simulink library "avlAero2DCoeffs_ul"  (R2018b)
settings: Solver=VariableStepAuto  StartTime=0.0  StopTime=10.0  RelTol=1e-3
values from neighbouring files (symbols this model uses):
  k_CS_gain = calculate_2D_gains(dsgnTest_1,nom_a,nom_b,df,da,de,dr)    [avlAero2DCoeffs_ts.m]
undefined symbols (not defined in the file or in its folder): CDtot_2D_Tbl, CLtot_2D_Tbl, Cltot_2D_Tbl, Cmtot_2D_Tbl, Cntot_2D_Tbl
settings Model: Creator=mcobb  LastModifiedBy=asiddiq2

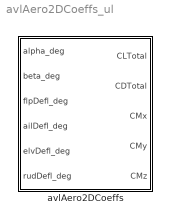
== system avlAero2DCoeffs_ul ==
  avlAero2DCoeffs : Subsystem  mask{CLTable=CLtot_2D_Tbl, CDTable=CDtot_2D_Tbl, CMxTable=Cltot_2D_Tbl, CMyTable=Cmtot_2D_Tbl, CMzTable=Cntot_2D_Tbl, CsGainMatrix=k_CS_gain}
      mask prompts: CLTable "CL lookup table object"; CDTable "CD lookup table object"; CMxTable "CMx lookup table object"; CMyTable "CMy lookup table object"; CMzTable "CMz lookup table object"; CsGainMatrix "Control surface gain matrix"

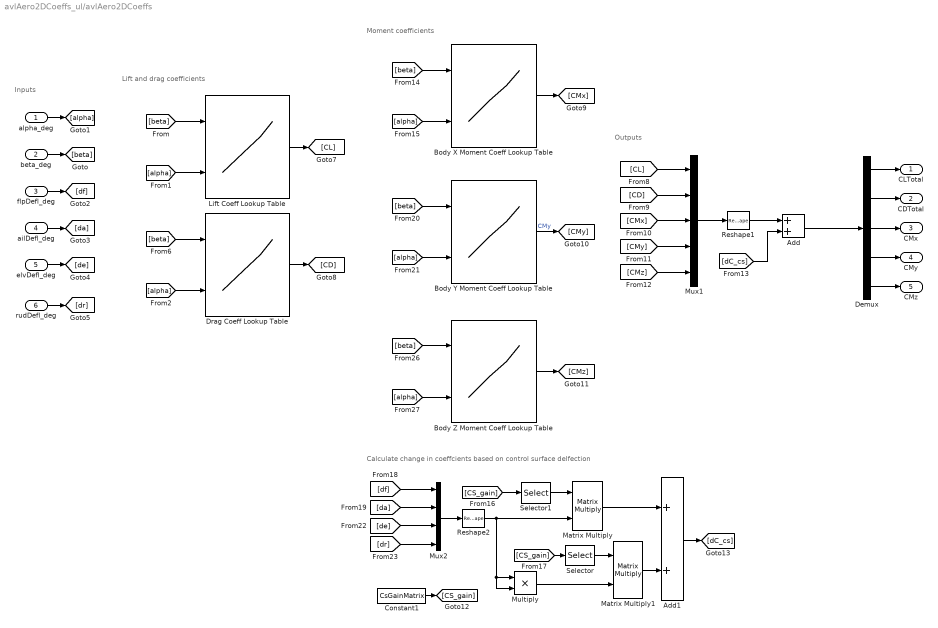
== system avlAero2DCoeffs_ul/avlAero2DCoeffs ==
  note: Outputs
  note: Inputs
  note: Lift and drag coefficients
  note: Moment coefficients
  note: Calculate change in coeffcients based on control surface
      | delfection
  alpha_deg : Inport
  beta_deg : Inport  Port=2
  flpDefl_deg : Inport  Port=3
  ailDefl_deg : Inport  Port=4
  elvDefl_deg : Inport  Port=5
  rudDefl_deg : Inport  Port=6
  Add : Sum
  Add1 : Sum
  Body X Moment Coeff Lookup Table : Lookup_n-D  DataSpecification=Lookup table object  LookupTableObject=CMxTable  BreakpointsForDimension3=[5, 7]  Table=reshape(repmat([4 5 6;16 19 20;10 18 23],1,2),[3,3,2])  InternalRulePriority=Speed  RndMeth=Simplest  InputSameDT=on
  Body Y Moment Coeff Lookup Table : Lookup_n-D  DataSpecification=Lookup table object  LookupTableObject=CMyTable  BreakpointsForDimension3=[5, 7]  Table=reshape(repmat([4 5 6;16 19 20;10 18 23],1,2),[3,3,2])  InternalRulePriority=Speed  RndMeth=Simplest  InputSameDT=on
  Body Z Moment Coeff Lookup Table : Lookup_n-D  DataSpecification=Lookup table object  LookupTableObject=CMzTable  BreakpointsForDimension3=[5, 7]  Table=reshape(repmat([4 5 6;16 19 20;10 18 23],1,2),[3,3,2])  InternalRulePriority=Speed  RndMeth=Simplest  InputSameDT=on
  Constant1 : Constant  Value=CsGainMatrix
  Demux : Demux  Outputs=5
  Drag Coeff Lookup Table : Lookup_n-D  DataSpecification=Lookup table object  LookupTableObject=CDTable  BreakpointsForDimension3=[5, 7]  Table=reshape(repmat([4 5 6;16 19 20;10 18 23],1,2),[3,3,2])  InternalRulePriority=Speed  RndMeth=Simplest  InputSameDT=on
  Lift Coeff Lookup Table : Lookup_n-D  DataSpecification=Lookup table object  LookupTableObject=CLTable  BreakpointsForDimension3=[5, 7]  Table=reshape(repmat([4 5 6;16 19 20;10 18 23],1,2),[3,3,2])  InternalRulePriority=Speed  RndMeth=Simplest  InputSameDT=on
  Matrix Multiply : Product  Multiplication=Matrix(*)
  Matrix Multiply1 : Product  Multiplication=Matrix(*)
  Multiply : Product
  Mux1 : Mux  Inputs=5
  Mux2 : Mux
  Reshape1 : Reshape  OutputDimensionality=Column vector (2-D)
  Reshape2 : Reshape  OutputDimensionality=Column vector (2-D)
  Selector : Selector  NumberOfDimensions=3  InputPortWidth=3  IndexOptions=Select all,Select all,Index vector (dialog)  Indices=[1 3],1,1  OutputSizes=1,1,1
  Selector1 : Selector  NumberOfDimensions=3  InputPortWidth=3  IndexOptions=Select all,Select all,Index vector (dialog)  Indices=[1 3],1,2  OutputSizes=1,1,1
  CLTotal : Outport
  CDTotal : Outport  Port=2
  CMx : Outport  Port=3
  CMy : Outport  Port=4
  CMz : Outport  Port=5
  wires:
  flpDefl_deg/1 -> [df]
  ailDefl_deg/1 -> [da]
  elvDefl_deg/1 -> [de]
  rudDefl_deg/1 -> [dr]
  [alpha] -> Lift Coeff Lookup Table/2
  [beta] -> Lift Coeff Lookup Table/1
  [beta] -> Drag Coeff Lookup Table/1
  [alpha] -> Drag Coeff Lookup Table/2
  [beta] -> Body X Moment Coeff Lookup Table/1
  [alpha] -> Body Z Moment Coeff Lookup Table/2
  [alpha] -> Body X Moment Coeff Lookup Table/2
  [beta] -> Body Z Moment Coeff Lookup Table/1
  [alpha] -> Body Y Moment Coeff Lookup Table/2
  [beta] -> Body Y Moment Coeff Lookup Table/1
  Lift Coeff Lookup Table/1 -> [CL]
  Drag Coeff Lookup Table/1 -> [CD]
  Body X Moment Coeff Lookup Table/1 -> [CMx]
  Body Y Moment Coeff Lookup Table/1 -> [CMy]  "CMy"
  Body Z Moment Coeff Lookup Table/1 -> [CMz]
  [CMx] -> Mux1/3
  [CL] -> Mux1/1
  [CD] -> Mux1/2
  [CMy] -> Mux1/4
  [CMz] -> Mux1/5
  Mux1/1 -> Reshape1/1
  Reshape1/1 -> Add/1
  [dC_cs] -> Add/2
  Add/1 -> Demux/1
  Demux/2 -> CDTotal/1
  Demux/1 -> CLTotal/1
  Demux/3 -> CMx/1
  Demux/4 -> CMy/1
  Demux/5 -> CMz/1
  beta_deg/1 -> [beta]
  alpha_deg/1 -> [alpha]
  Multiply/1 -> Matrix Multiply1/2
  Matrix Multiply1/1 -> Add1/2
  Matrix Multiply/1 -> Add1/1
  Reshape2/1 -> Multiply/2, Multiply/1, Matrix Multiply/2
  Add1/1 -> [dC_cs]
  [df] -> Mux2/1
  Selector1/1 -> Matrix Multiply/1
  [CS_gain] -> Selector1/1
  Selector/1 -> Matrix Multiply1/1
  Constant1/1 -> [CS_gain]
  [CS_gain] -> Selector/1
  [da] -> Mux2/2
  [dr] -> Mux2/4
  Mux2/1 -> Reshape2/1
  [de] -> Mux2/3
